simulink model "TestDUE_SineWave"  (R2019b)
settings: Solver=FixedStepDiscrete  StartTime=0.0  StopTime=inf  FixedStep=50e-6  RelTol=1e-3  EnableMultiTasking=on
libraries: arduinolib x1
settings Model: SimulationMode=external  ExtModeTrigDuration=2  Creator=Marta Nohemi Montalvo  LastModifiedBy=F Gonzalez-Longatt
settings Model: ModifiedHistory=|
  | Created: Angel Barrios, UK 2018
  | Improved and modified: Marta Nohemi Montalvo
  | Supervised: Prof Francisco Gonzalez-Longatt
settings DataIOCC: ReturnWorkspaceOutputs=off
settings OptimizationCC: EnhancedBackFolding=on  PassReuseOutputArgsAs=Individual arguments  MaxStackSize=64  OptimizeBlockOrder=speed  DifferentSizesBufferReuse=on  OptimizationCustomize=off  EfficientTunableParamExpr=on
settings DebuggingCC: ParameterTunabilityLossMsg=error  ArithmeticOperatorsInVariantConditions=warning
settings HardwareCC: ProdBitPerPointer=32  ProdBitPerSizeT=32  ProdBitPerPtrDiffT=32  ProdLargestAtomicInteger=Long  ProdLargestAtomicFloat=Double  ProdWordSize=32  ProdHWDeviceType=ARM Compatible->ARM Cortex
settings SFSimCC: MATLABDynamicMemAlloc=off  CustomCodeUndefinedFunction=UseInterfaceOnly
settings RTWCC: SystemTargetFile=ert.tlc  HardwareBoard=Arduino Due  TLCOptions=-aInlineSetEventsForThisBaseRateFcn=TLC_FALSE -aSuppressMultiTaskScheduler=TLC_FALSE -aRateBasedStepFcn=1  TemplateMakefile=ert_default_tmf  GenerateReport=on  Toolchain=Arduino ARM  BuildConfiguration=Faster Runs  IncludeHyperlinkInReport=on  LaunchReport=on  GenerateTraceInfo=on  GenerateTraceReport=on  GenerateTraceReportSl=on  GenerateTraceReportSf=on  GenerateTraceReportEml=on
settings CodeAppCC: ForceParamTrailComments=on  IgnoreCustomStorageClasses=off  OperatorAnnotations=on  SimulinkDataObjDesc=on  SFDataObjDesc=on  InsertBlockDesc=on
settings ERTTargetCC: SupportContinuousTime=on  SupportVariableSizeSignals=on

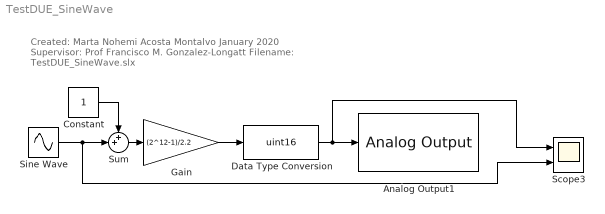
== system TestDUE_SineWave ==
  note: Created: Marta Nohemi Acosta Montalvo January 2020
      | Supervisor: Prof Francisco M. Gonzalez-Longatt
      | Filename: TestDUE_SineWave.slx
  Analog Output1 : arduinolib/Analog Output  DACpin=DAC0  blockPlatform=arduino
      settings: SourceProductName=Simulink Support Package for Arduino Hardware  SourceProductBaseCode=ARDUINO
  Constant : Constant
  Data Type Conversion : DataTypeConversion  OutDataTypeStr=uint16
  Gain : Gain  Gain=(2^12-1)/2.2
  Scope3 : Scope  NumInputPorts=2
  Sine Wave : Sin  Frequency=314.1593  SampleTime=0
  Sum : Sum  Inputs=++|
  wires:
  Gain/1 -> Data Type Conversion/1
  Sine Wave/1 -> Sum/2, Scope3/2
  Sum/1 -> Gain/1
  Data Type Conversion/1 -> Analog Output1/1, Scope3/1
  Constant/1 -> Sum/1
